simulink model "r_axis_plant"  (R2024b)
settings: Solver=ode45  StartTime=0.0  StopTime=simulation_time  MaxStep=1e-3  RelTol=1e-8  AbsTol=1e-10
undefined symbols (not defined in the file): b_r, F_test, m_r, r_initial
settings Model: Creator=dell  LastModifiedBy=dell

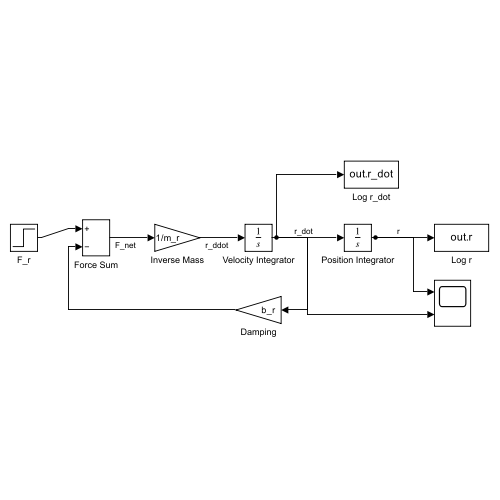
[thumbnail: Simulink's stored preview of the top-level diagram]
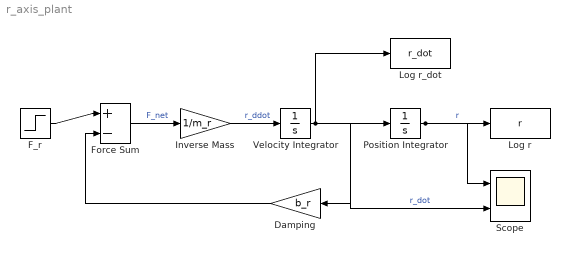
== system r_axis_plant ==
  Damping : Gain  Gain=b_r
  F_r : Step  Time=0  After=F_test  SampleTime=0
  Force Sum : Sum  Inputs=+-
  Inverse Mass : Gain  Gain=1/m_r
  Log r : ToWorkspace  VariableName=r  SaveFormat=Timeseries  SampleTime=-1
  Log r_dot : ToWorkspace  VariableName=r_dot  SaveFormat=Timeseries  SampleTime=-1
  Position Integrator : Integrator  InitialCondition=r_initial
  Scope : Scope  NumInputPorts=2
  Velocity Integrator : Integrator
  wires:
  F_r/1 -> Force Sum/1
  Force Sum/1 -> Inverse Mass/1  "F_net"
  Inverse Mass/1 -> Velocity Integrator/1  "r_ddot"
  Velocity Integrator/1 -> Position Integrator/1, Damping/1, Log r_dot/1, Scope/2  "r_dot"
  Damping/1 -> Force Sum/2
  Position Integrator/1 -> Log r/1, Scope/1  "r"
